simulink model "mcb_microchip_pmsm_foc_sensorless_SAME70"  (R2021b)
settings: Solver=FixedStepDiscrete  StartTime=0.0  StopTime=5  FixedStep=Ts/2  RelTol=1e-3  EnableMultiTasking=on
InitFcn:
  | mcb_microchip_pmsm_foc_sensorless_SAME70_data
values from neighbouring files (symbols this model uses):
  PI_params = mcb.internal.SetControllerParameters(pmsm,inverter,PU_System,T_pwm,2*Ts,Ts_speed)    [mcb_microchip_pmsm_foc_sensorless_SAME70_data.m]
  PU_System = mcb_SetPUSystem(pmsm,inverter)    [mcb_microchip_pmsm_foc_sensorless_SAME70_data.m]
  PWM_frequency = 20e3    (= 20000)    [mcb_microchip_pmsm_foc_sensorless_SAME70_data.m]
  Ts = T_pwm    (= 5e-05)    [mcb_microchip_pmsm_foc_sensorless_SAME70_data.m]
  Ts_motor = T_pwm/2    (= 2.5e-05)    [mcb_microchip_pmsm_foc_sensorless_SAME70_data.m]
  Ts_simulink = T_pwm/2    (= 2.5e-05)    [mcb_microchip_pmsm_foc_sensorless_SAME70_data.m]
  Ts_speed = 20*Ts    (= 0.001)    [mcb_microchip_pmsm_foc_sensorless_SAME70_data.m]
  Vd_Ref_openLoop_PU = 0.1    [mcb_microchip_pmsm_foc_sensorless_SAME70_data.m]
undefined symbols (not defined in the file or in its folder): A24, AD10, AD7, DiscIntNeverNeededParam, inverter, LQFP144, PA10, PA11, PA12, PA13, PA18, PA9, PB0, PD18, PD19, PD24, PD25, PD26, Pin, pmsm, SAME70Q21B, Timer, Unsigned
libraries: mcbcontrolslib x15, simulink x15, MCHP_Blockset x11, mcbpositiondecoderlib x3, mcbsensorlessestimatorlib x1, mcbplantlib x1, autolibpmsmexterior x1
(part 4 of 4)

== system mcb_microchip_pmsm_foc_sensorless_SAME70/Current Control/Input Scaling/Calculate position and speed/Sliding Mode Observer ==
  InputSignals : Inport
  Action Port : ActionPort  ActionPortLabel=case [ 0 ]:
  Data Store Read1 : DataStoreRead  DataStoreName=Enable  IndexOptions=Index vector (dialog)  Indices=1  OutputSizes=1
  Demux1 : Demux
  Logical Operator : Logic  Operator=NOT  IconShape=distinctive  AllPortsSameDT=off  OutDataTypeStr=boolean
  Mux : Mux  Inputs=2
  Sliding Mode Observer : mcbsensorlessestimatorlib/Sliding Mode Observer  InputUnit=Per-unit  BlkSampleTime=Ts  StatorResistance=pmsm.Rs  StatorInductance=pmsm.Ld  MaxApplicationSpeed=pmsm.N_base  PolePairs=pmsm.p  MaxStatorVoltage=PU_System.V_base  MaxStatorCurrent=PU_System.I_base  DisturbanceObserverGain=smo.BackEmfObsGain  CurrentObserverGain=smo.CurrentObsGain  CutoffFreq=smo.CutoffFreq  PositionUnit=Per unit  PositionDataType=dataType  SpeedUnit=Per unit  PerUnitSpeed=PU_System.N_base  SpeedDataType=dataType
      settings: SourceProductBaseCode=MT
  Position/Speed : Outport
  wires:
  Mux/1 -> Position/Speed/1
  Demux1/1 -> Sliding Mode Observer/1
  Demux1/2 -> Sliding Mode Observer/2
  Demux1/4 -> Sliding Mode Observer/4  "Ibeta"
  Demux1/3 -> Sliding Mode Observer/3  "Ialpha"
  Sliding Mode Observer/1 -> Mux/1
  Sliding Mode Observer/2 -> Mux/2
  InputSignals/1 -> Demux1/1
  Data Store Read1/1 -> Logical Operator/1
  Logical Operator/1 -> Sliding Mode Observer/5

== system mcb_microchip_pmsm_foc_sensorless_SAME70/Current Control/Output Scaling/Mode Selector/Subsystem1 ==
  Count : Inport
  Compare To Constant : simulink/Logic and Bit Operations/Compare To Constant  relop=>=  const=2  OutDataTypeStr=boolean
  Compare To Constant1 : simulink/Logic and Bit Operations/Compare To Constant  relop=<  const=1  OutDataTypeStr=boolean
  Data Store Write : DataStoreWrite  DataStoreName=EnCurOffset  IndexOptions=Index vector (dialog)  Indices=1  OutputSizes=1
  Gain : Gain  Gain=1/(PWM_frequency)  OutDataTypeStr=dataType  RndMeth=Simplest
  Current Offset : Outport
  EnClosedLoop : Outport  Port=2
  wires:
  Count/1 -> Gain/1
  Gain/1 -> Compare To Constant1/1, Compare To Constant/1
  Compare To Constant/1 -> EnClosedLoop/1
  Compare To Constant1/1 -> Data Store Write/1, Current Offset/1

== system mcb_microchip_pmsm_foc_sensorless_SAME70/Current Control/Output Scaling/Mode Selector/Up Counter ==
  Enable : EnablePort
  Add1 : Sum  SaturateOnIntegerOverflow=on
  Constant : Constant  OutDataTypeStr=uint32
  Delay : Delay  DelayLength=1
  Count : Outport  InitialOutput=0
  wires:
  Delay/1 -> Add1/2
  Add1/1 -> Count/1, Delay/1
  Constant/1 -> Add1/1

== system mcb_microchip_pmsm_foc_sensorless_SAME70/Inverter and Motor - Plant Model/Plant Model/Inverter and Motor (sim)/Inverter ==
  Duty_abc : Inport
  Average-Value Inverter : mcbplantlib/Average-Value Inverter
  Constant2 : Constant  Value=inverter.V_dc  OutDataTypeStr=single  SampleTime=-1
  Data Type Conversion1 : DataTypeConversion  OutDataTypeStr=single  RndMeth=Simplest
  Rate Transition3 : RateTransition  Deterministic=off  OutPortSampleTime=Ts_inverter
  Vabc : Outport  VectorParamsAs1DForOutWhenUnconnected=off
  wires:
  Constant2/1 -> Average-Value Inverter/2
  Data Type Conversion1/1 -> Rate Transition3/1
  Duty_abc/1 -> Data Type Conversion1/1
  Average-Value Inverter/1 -> Vabc/1
  Rate Transition3/1 -> Average-Value Inverter/1

== system mcb_microchip_pmsm_foc_sensorless_SAME70/Inverter and Motor - Plant Model/Plant Model/Inverter and Motor (sim)/Load_Profile (Torque) ==
  Data Type Conversion : DataTypeConversion  OutDataTypeStr=single
  IIR Filter : mcbcontrolslib/IIR Filter  VariantControl=Low Pass Filter  VariantSelect=Low-pass  Filter_constant=0.0001  advancedSettings=off  Ts=50e-6  cutOff_freq=0.31834
      settings: SourceProductBaseCode=MT
  T_load : Step  Time=3  Before=0*pmsm.T_rated  After=0.5*pmsm.T_rated  SampleTime=Ts_simulink
  Load_Trq : Outport  VectorParamsAs1DForOutWhenUnconnected=off
  wires:
  Data Type Conversion/1 -> IIR Filter/1
  IIR Filter/1 -> Load_Trq/1
  T_load/1 -> Data Type Conversion/1

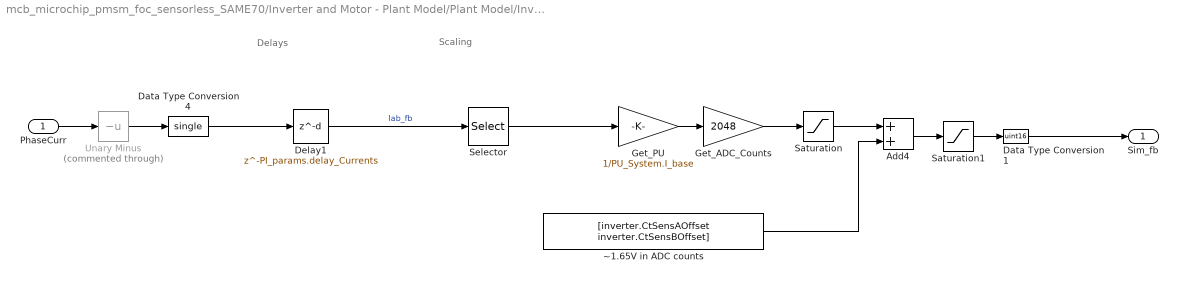
== system mcb_microchip_pmsm_foc_sensorless_SAME70/Inverter and Motor - Plant Model/Plant Model/Inverter and Motor (sim)/Sensor_Measurements ==
  note: Scaling
  note: Delays
  PhaseCurr : Inport
  Add4 : Sum  OutDataTypeStr=uint16
  Data Type Conversion1 : DataTypeConversion  OutDataTypeStr=uint16
  Data Type Conversion4 : DataTypeConversion  OutDataTypeStr=single  RndMeth=Simplest
  Delay1 : Delay  DelayLength=PI_params.delay_Currents
  Get_ADC_Counts : Gain  Gain=2048  RndMeth=Simplest  OutDataTypeStr=Inherit: Same as input
  Get_PU : Gain  Gain=1/PU_System.I_base  RndMeth=Simplest
  Saturation : Saturate  UpperLimit=2048  LowerLimit=-2048
  Saturation1 : Saturate  UpperLimit=4095  LowerLimit=0
  Selector : Selector  InputPortWidth=3  IndexOptions=Index vector (dialog)  Indices=[1 2]  OutputSizes=1
  Unary Minus : UnaryMinus  Commented=through
  ~1.65V in ADC counts : Constant  Value=[inverter.CtSensAOffset inverter.CtSensBOffset]  OutDataTypeStr=uint16  SampleTime=-1
  Sim_fb : Outport  VectorParamsAs1DForOutWhenUnconnected=off
  wires:
  Get_ADC_Counts/1 -> Saturation/1
  Saturation1/1 -> Data Type Conversion1/1
  Add4/1 -> Saturation1/1
  ~1.65V in ADC counts/1 -> Add4/2
  Delay1/1 -> Selector/1  "Iab_fb"
  Saturation/1 -> Add4/1
  Data Type Conversion4/1 -> Delay1/1
  PhaseCurr/1 -> Unary Minus/1
  Get_PU/1 -> Get_ADC_Counts/1
  Data Type Conversion1/1 -> Sim_fb/1
  Selector/1 -> Get_PU/1
  Unary Minus/1 -> Data Type Conversion4/1

== system mcb_microchip_pmsm_foc_sensorless_SAME70/Serial Receive/CodeGen/Subsystem/unParse ==
  Data : Inport
  Bitwise Operator : simulink/Logic and Bit Operations/Bitwise Operator  logicop=AND  UseBitMask=on  BitMask=hex2dec('0001')  BitMaskRealWorld=Stored Integer
  Bitwise Operator1 : simulink/Logic and Bit Operations/Bitwise Operator  logicop=AND  UseBitMask=on  BitMask=hex2dec('00F0')  BitMaskRealWorld=Stored Integer
  Data Type Conversion3 : DataTypeConversion  OutDataTypeStr=boolean  RndMeth=Simplest
  Data Type Conversion4 : DataTypeConversion  OutDataTypeStr=uint16  RndMeth=Simplest
  Shift Arithmetic1 : ArithShift  BitShiftNumber=4
  Enable_PWM : Outport
  Debug_signals : Outport  Port=2
  wires:
  Bitwise Operator1/1 -> Shift Arithmetic1/1
  Data/1 -> Bitwise Operator/1, Bitwise Operator1/1
  Bitwise Operator/1 -> Data Type Conversion3/1
  Data Type Conversion4/1 -> Debug_signals/1
  Shift Arithmetic1/1 -> Data Type Conversion4/1
  Data Type Conversion3/1 -> Enable_PWM/1

== system mcb_microchip_pmsm_foc_sensorless_SAME70/Serial Receive/CodeGen/Subsystem1/Triggered Subsystem ==
  In1 : Inport
  Enable : EnablePort
  Data out : Outport
  wires:
  In1/1 -> Data out/1

== system mcb_microchip_pmsm_foc_sensorless_SAME70/Current Control/Closed Loop/Open_Loop_Control/Check actual speed/Subsystem ==
  In1 : Inport
  Enable : EnablePort
  Compare To Constant1 : simulink/Logic and Bit Operations/Compare To Constant  relop=>  const=Vd_Ref_openLoop_PU * 0.95  OutDataTypeStr=boolean
  Output : Outport
  wires:
  In1/1 -> Compare To Constant1/1
  Compare To Constant1/1 -> Output/1

== system mcb_microchip_pmsm_foc_sensorless_SAME70/Current Control/Input Scaling/Calculate position and speed/Flux Observer/high_pass_filter ==
  In1 : Inport
  IIR Filter1 : mcbcontrolslib/IIR Filter  VariantControl=Low Pass Filter  VariantSelect=Low-pass  Filter_constant=0.001  advancedSettings=off  Ts=50e-6  cutOff_freq=3.1863
      settings: SourceProductBaseCode=MT
  Sum : Sum  Inputs=|+-  OutDataTypeStr=Inherit: Same as first input
  Out1 : Outport
  wires:
  In1/1 -> IIR Filter1/1, Sum/1
  IIR Filter1/1 -> Sum/2
  Sum/1 -> Out1/1
